simulink subsystem "matrixDeterminant"  (R2024b)
settings: Solver=VariableStepAuto  StartTime=0.0  StopTime=10.0  RelTol=1e-3
settings Model: Creator=ricca  LastModifiedBy=ricca

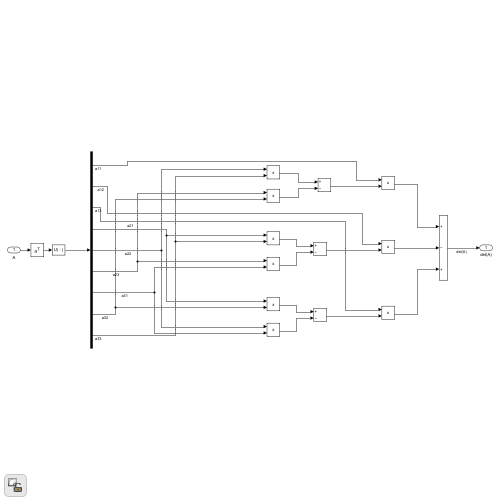
[thumbnail: Simulink's stored preview of the top-level diagram]
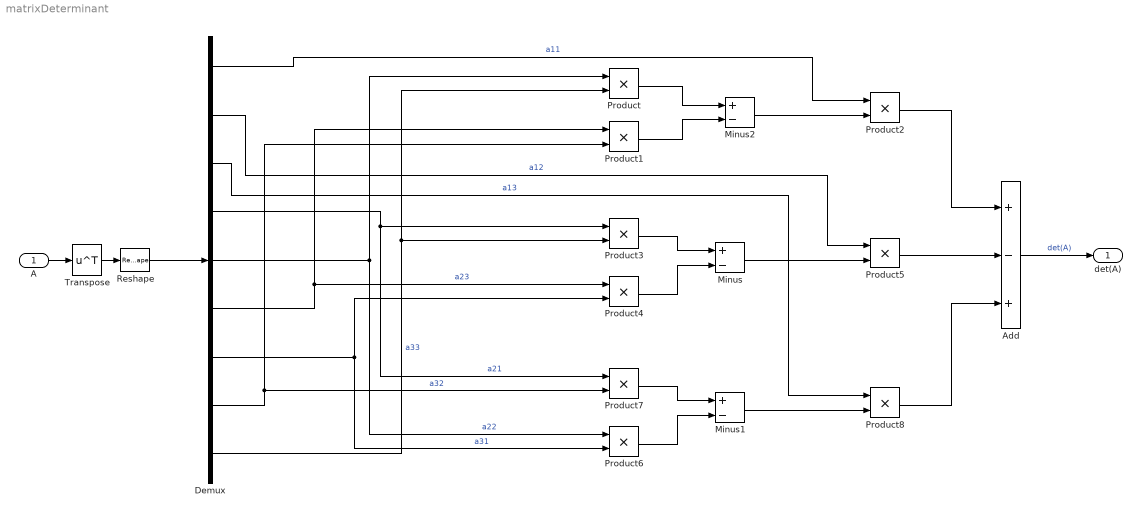
== system matrixDeterminant ==
  A : Inport
  Add : Sum  Inputs=+-+
  Demux : Demux  Outputs=9
  Minus : Sum  Inputs=+-
  Minus1 : Sum  Inputs=+-
  Minus2 : Sum  Inputs=+-
  Product{,1..8} (9 alike) : Product
  Reshape : Reshape
  Transpose : Math  Operator=transpose
  det(A) : Outport
  wires:
  A/1 -> Transpose/1
  Demux/3 -> Product8/1  "a13"
  Demux/4 -> Product3/1, Product7/1  "a21"
  Demux/5 -> Product/1, Product6/1  "a22"
  Minus2/1 -> Product2/2
  Add/1 -> det(A)/1  "det(A)"
  Product7/1 -> Minus1/1
  Product4/1 -> Minus/2
  Product6/1 -> Minus1/2
  Product1/1 -> Minus2/2
  Demux/9 -> Product/2, Product3/2  "a33"
  Demux/8 -> Product1/2, Product7/2  "a32"
  Minus/1 -> Product5/2
  Demux/2 -> Product5/1  "a12"
  Demux/7 -> Product6/2, Product4/2  "a31"
  Demux/6 -> Product1/1, Product4/1  "a23"
  Minus1/1 -> Product8/2
  Product5/1 -> Add/2
  Product2/1 -> Add/1
  Product3/1 -> Minus/1
  Product/1 -> Minus2/1
  Demux/1 -> Product2/1  "a11"
  Product8/1 -> Add/3
  Reshape/1 -> Demux/1
  Transpose/1 -> Reshape/1
